simulink model "feedback_plant"  (R2016a)
settings: Solver=FixedStepAuto  StartTime=0.0  StopTime=9660  MaxStep=0.1  RelTol=1e-3
undefined symbols (not defined in the file): sensors
libraries: slrtlib x8, xpcnilib x2, simulink x2
settings Model: ModifiedByFormat=The MathWorks Inc.  Creator=The MathWorks, Inc.  LastModifiedBy=The MathWorks Inc.
settings SolverCC: EnableConcurrentExecution=on
settings DataIOCC: LimitDataPoints=on  SaveFormat=Array
settings OptimizationCC: BlockReduction=off  DefaultParameterBehavior=Inlined  OptimizeBlockIOStorage=off  BufferReuse=off  GlobalBufferReuse=off  ExpressionFolding=off  ExpressionDepthLimit=2147483647  LocalBlockOutputs=off
settings DebuggingCC: UnderspecifiedInitializationDetection=Classic  MergeDetectMultiDrivingBlocksExec=none  SolverPrmCheckMsg=warning  FcnCallInpInsideContextMsg=EnableAllAsWarning  AllowSymbolicDim=off  StateNameClashWarn=warning
settings HardwareCC: ProdBitPerPointer=32  ProdLargestAtomicFloat=None  ProdWordSize=32  ProdLongLongMode=on  ProdHWDeviceType=Generic->32-bit x86 compatible
settings ModelReferenceCC: ModelReferenceNumInstancesAllowed=Single  ModelReferenceMinAlgLoopOccurrences=on  PropagateSignalLabelsOutOfModel=off
settings RTWCC: SystemTargetFile=slrt.tlc  TemplateMakefile=slrt_default_tmf  Description=Simulink Real-Time  RTWVerbose=off
settings ConfigComp: CovModelRefEnable=Off  CovSFcnEnable=off

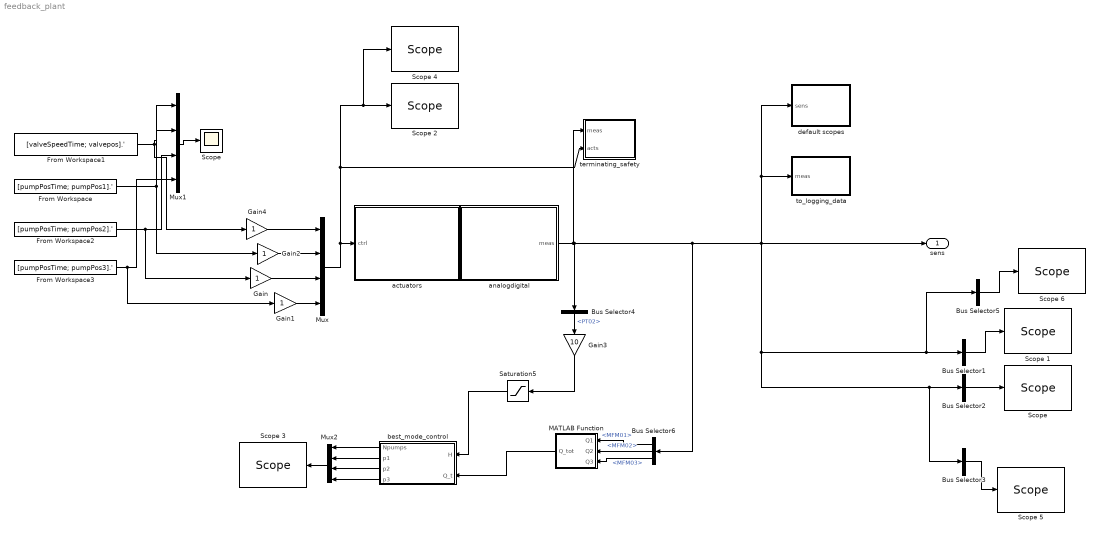
== system feedback_plant ==
  Bus Selector1 : BusSelector  OutputSignals=CV01,DPT01,DPT02,DPT03,MFM01,MFM02,MFM03,PT02  OutputAsBus=on
  Bus Selector2 : BusSelector  OutputSignals=LMGV1,LMGV2,LMGV3,LMGC1,LMGC2,LMGC3,LMGP1,LMGP2,LMGP3  OutputAsBus=on
  Bus Selector3 : BusSelector  OutputSignals=WP01,WP02,WP03  OutputAsBus=on
  Bus Selector4 : BusSelector  OutputSignals=PT02
  Bus Selector5 : BusSelector  OutputSignals=PT02  OutputAsBus=on
  Bus Selector6 : BusSelector  OutputSignals=MFM01,MFM02,MFM03
  From Workspace : FromWorkspace  VariableName=[pumpPosTime; pumpPos1].'  SampleTime=0  Interpolate=off  OutputAfterFinalValue=Holding final value
  From Workspace1 : FromWorkspace  VariableName=[valveSpeedTime; valvepos].'  SampleTime=0  Interpolate=off  OutputAfterFinalValue=Holding final value
  From Workspace2 : FromWorkspace  VariableName=[pumpPosTime; pumpPos2].'  SampleTime=0  Interpolate=off  OutputAfterFinalValue=Holding final value
  From Workspace3 : FromWorkspace  VariableName=[pumpPosTime; pumpPos3].'  SampleTime=0  Interpolate=off  OutputAfterFinalValue=Holding final value
  Gain{,1..2,4} (4 alike) : Gain
  Gain3 : Gain  Gain=10
  MATLAB Function : MATLAB Function  TreatAsAtomicUnit=on
  Mux : Mux
  Mux1 : Mux
  Mux2 : Mux
  Saturation5 : Saturate  UpperLimit=200  LowerLimit=0.001
  Scope : Scope
  "Scope " : slrtlib/Displays and Logging/Scope   scopeno=9  scopetype=Target  autostart=on  viewmode=Numerical  formatstr='%15.6f'  grid=on  ylimits=[0,0]  nosamples=25  noprepostsamples=0  interleave=1  triggermode=FreeRun  triggersignal=1  trigsignalfromport=off  triggerlevel=0.0  triggerslope=Either  triggerscope=1  triggersample=0  filename=data.dat  mode=Lazy  writesize=512  autorestart=off  dynamicfilemode=off  maxwritefilesize=512*1024^2
  Scope 1 : slrtlib/Displays and Logging/Scope   scopeno=10  scopetype=Target  autostart=on  viewmode=Numerical  formatstr='%15.6f'  grid=on  ylimits=[0,0]  nosamples=25  noprepostsamples=0  interleave=1  triggermode=FreeRun  triggersignal=1  trigsignalfromport=off  triggerlevel=0.0  triggerslope=Either  triggerscope=1  triggersample=0  filename=data.dat  mode=Lazy  writesize=512  autorestart=off  dynamicfilemode=off  maxwritefilesize=512*1024^2
  Scope 2 : slrtlib/Displays and Logging/Scope   scopeno=2  scopetype=Host  autostart=on  viewmode=Graphical redraw  formatstr='%15.6f'  grid=on  ylimits=[0,0]  nosamples=250  noprepostsamples=0  interleave=1  triggermode=FreeRun  triggersignal=1  trigsignalfromport=off  triggerlevel=0.0  triggerslope=Either  triggerscope=1  triggersample=0  filename=data.dat  mode=Lazy  writesize=512  autorestart=off  dynamicfilemode=off  maxwritefilesize=512*1024^2
  Scope 3 : slrtlib/Displays and Logging/Scope   scopeno=3  scopetype=Host  autostart=on  viewmode=Graphical redraw  formatstr='%15.6f'  grid=on  ylimits=[0,0]  nosamples=250  noprepostsamples=0  interleave=1  triggermode=FreeRun  triggersignal=1  trigsignalfromport=off  triggerlevel=0.0  triggerslope=Either  triggerscope=1  triggersample=0  filename=data.dat  mode=Lazy  writesize=512  autorestart=off  dynamicfilemode=off  maxwritefilesize=512*1024^2
  Scope 4 : slrtlib/Displays and Logging/Scope   scopeno=8  scopetype=Target  autostart=on  viewmode=Numerical  formatstr='%15.6f'  grid=on  ylimits=[0,0]  nosamples=25  noprepostsamples=0  interleave=1  triggermode=FreeRun  triggersignal=1  trigsignalfromport=off  triggerlevel=0.0  triggerslope=Either  triggerscope=1  triggersample=0  filename=data.dat  mode=Lazy  writesize=512  autorestart=off  dynamicfilemode=off  maxwritefilesize=512*1024^2
  Scope 5 : slrtlib/Displays and Logging/Scope   scopeno=11  scopetype=Target  autostart=on  viewmode=Numerical  formatstr='%15.6f'  grid=on  ylimits=[0,0]  nosamples=25  noprepostsamples=0  interleave=1  triggermode=FreeRun  triggersignal=1  trigsignalfromport=off  triggerlevel=0.0  triggerslope=Either  triggerscope=1  triggersample=0  filename=data.dat  mode=Lazy  writesize=512  autorestart=off  dynamicfilemode=off  maxwritefilesize=512*1024^2
  Scope 6 : slrtlib/Displays and Logging/Scope   scopeno=4  scopetype=Target  autostart=on  viewmode=Graphical sliding  formatstr='%15.6f'  grid=on  ylimits=[0,0]  nosamples=100  noprepostsamples=0  interleave=1  triggermode=FreeRun  triggersignal=1  trigsignalfromport=off  triggerlevel=0.0  triggerslope=Either  triggerscope=1  triggersample=0  filename=data.dat  mode=Lazy  writesize=512  autorestart=off  dynamicfilemode=off  maxwritefilesize=512*1024^2
  actuators : Subsystem  mask{actuators_list={'CV03', 'CV05'}, subsystem=[3,1]}
      mask init:
      | %%Get analog channels
      | actuators = evalin('base','actuators');
      | 
      | subsystem = sprintf('[%d,%d]', subsystem(1), subsystem(2));
      | 
      | %actuators = actuators(strcmp(subsystem,{actuators.PCIslot}));
      | 
      | src_block = find_system(gcb, 'LookUnderMasks', 'on','Name', 'DA_sink');
      | maskObj = Simulink.Mask.get(src_block{1});
      | 
      | if(isempty(actuators))
      |    error('There are no analog outputs in the given card'); 
      | end
      | 
      | maskObj.Parameters(1,5).Value = subsystem;
      | maskObj.Parameters(1,1).Value = mat2str([actuators.Channel]+1);
      | Simulink.Block.eval(src_block{1});
      | 
      | %Find block
      | transform_blk = find_system(gcb, 'LookUnderMasks', 'on','Name', 'transform');
      | 
      | outputnames = {actuators.Name};
      | outputs = strjoin(outputnames,',');
      | 
      | sigcount = numel(outputnames);
      | sigstring = num2str(sigcount);
      | 
      | %Transform block
      | transform_blk = find_system(gcb, 'LookUnderMasks', 'on','Name', 'transform');
      | lines{1}=['function [' outputs ']  = fcn(u,gain,offset)'];
      | lines{2}='   y = u.*gain-offset;';
      | for i=1:numel(outputnames)
      |    %start at 4
      |    lines{2+i} = [ outputnames{i} ' = y(' num2str(i) ');'];
      | end
      | outputscript = strjoin(lines,'\n');
      | matlabfunctionfromstring(transform_blk{1}, outputscript);
      | Simulink.Block.eval(transform_blk{1});
      | 
      | %Delete lines
      | connections = find_system(gcb,'findall','on','LookUnderMasks', 'on','SearchDepth', 1,'type','line');
      | delete_line(connections);
      | 
      | for i=1:numel(outputnames)
      |    add_line(gcb,['transform/' num2str(i) ],['DA_sink/' num2str(i)],'autorouting','on');
      | end
      | 
      | %Transform block
      | add_line(gcb,'ctrl/1','transform/1','autorouting','on')
      | add_line(gcb,'gain/1','transform/2','autorouting','on')
      | add_line(gcb,'offset/1','transform/3','autorouting','on')
      | 
      | gain = [actuators.Gain]';
      | offset = [actuators.Offset]';
  analogdigital : Subsystem  mask{gain=[sensors.Gain], offset=[sensors.Offset]}
      mask init:
      | %%Get analog channels
      | sensors = evalin('base','sensors');
      | 
      | %subsystem = sprintf('[%d,%d]', subsystem(1), subsystem(2));
      | 
      | %analogin = sensors(strcmp(subsystem,{sensors.PCIslot})&(strcmp('VI|0-10V',{sensors.Type})|strcmp('VI|2-10V',{sensors.Type})|strcmp('CI|4-20mA',{sensors.Type})));
      | if ~isempty(sensors)
      | %    disp(['PCI slot ' subsystem ' loading']);
      | else
      |     error('There are no analog inputs in the given card'); 
      | end
      | 
      | 
      | %%Find source (ADC) block
      | src_block = find_system(gcb, 'LookUnderMasks', 'on','Name', 'src');
      | maskObj = Simulink.Mask.get(src_block{1});
      | 
      | %maskObj.Parameters(1,6).Value = subsystem;
      | maskObj.Parameters(1,1).Value = mat2str([sensors.Channel]+1);
      | Simulink.Block.eval(src_block{1});
      | 
      | %Find block
      | transform_blk = find_system(gcb, 'LookUnderMasks', 'on','Name', 'transform');
      | 
      | outputnames = {sensors.Name};
      | outputs = strjoin(outputnames,',');
      | 
      | sigcount = numel(outputnames);
      | sigstring = num2str(sigcount);
      | 
      | %Transform block
      | transform_blk = find_system(gcb, 'LookUnderMasks', 'on','Name', 'transform');
      | lines{1}=['function [' outputs ']  = fcn(u,gain,offset)'];
      | lines{2}='   y = u(:).*gain(:)-offset(:);';
      | for i=1:numel(outputnames)
      |    %start at 4
      |    lines{2+i} = [ outputnames{i} ' = y(' num2str(i) ');'];
      | end
      | outputscript = strjoin(lines,'\n');
      | matlabfunctionfromstring(transform_blk{1}, outputscript);
      | Simulink.Block.eval(transform_blk{1});
      | 
      | %Delete lines
      | connections = find_system(gcb,'findall','on','LookUnderMasks', 'on','SearchDepth', 1,'type','line');
      | delete_line(connections);
      | 
      | %Mux block
      | mux_blk = find_system(gcb, 'LookUnderMasks', 'on','Name', 'mux');
      | set_param(mux_blk{1},'Inputs', sigstring);
      | Simulink.Block.eval(mux_blk{1});
      | 
      | %Bus block
      | bus_blk = find_system(gcb, 'LookUnderMasks', 'on','Name', 'bus');
      | set_param(bus_blk{1},'Inputs', sigstring);
      | Simulink.Block.eval(bus_blk{1});
      | 
      | for i=1:numel(outputnames)
      |    add_line(gcb,['src/' num2str(i) ],['mux/' num2str(i)],'autorouting','on');
      |    add_line(gcb,['transform/' num2str(i) ],['bus/' num2str(i)],'autorouting','on');
      | end
      | 
      | %Lines to bus block
      | p = get_param(transform_blk, 'PortHandles');
      | l = get_param(p{1}.Outport,'Line');
      | 
      | for i=1:numel(outputnames)
      |    set_param(l{i},'Name',outputnames{i}) 
      | end
      | 
      | %Transform block
      | add_line(gcb,'mux/1','transform/1','autorouting','on')
      | add_line(gcb,'bus/1','meas/1','autorouting','on')
  best_mode_control : Subsystem
  default scopes : Subsystem
  terminating_safety : Subsystem
      mask init:
      | str1 = evalin('base', 'strjoin({sensors.Name},''/'')');
      | sensnames = uint8(str1);
  to_logging_data : Subsystem
  sens : Outport
  wires:
  Mux/1 -> actuators/1(ctrl), terminating_safety/2(acts), Scope 4/1, Scope 2/1
  Bus Selector2/1 -> "Scope "/1
  Bus Selector1/1 -> Scope 1/1
  Mux1/1 -> Scope/1
  From Workspace1/1 -> Mux1/1, Gain4/1
  From Workspace/1 -> Gain2/1, Mux1/2
  Bus Selector3/1 -> Scope 5/1
  Bus Selector5/1 -> Scope 6/1
  Gain/1 -> Mux/3
  Gain1/1 -> Mux/4
  Gain2/1 -> Mux/2
  analogdigital/1(meas) -> terminating_safety/1(meas), Bus Selector6/1, default scopes/1(sens), to_logging_data/1(meas), Bus Selector5/1, Bus Selector1/1, Bus Selector3/1, Bus Selector2/1, sens/1, Bus Selector4/1
  Bus Selector6/2 -> MATLAB Function/2(Q2)  "<MFM02>"
  Bus Selector6/1 -> MATLAB Function/1(Q1)  "<MFM01>"
  Bus Selector6/3 -> MATLAB Function/3(Q3)  "<MFM03>"
  MATLAB Function/1(Q_tot) -> best_mode_control/2(Q_t)
  Bus Selector4/1 -> Gain3/1  "<PT02>"
  Gain3/1 -> Saturation5/1
  Mux2/1 -> Scope 3/1
  best_mode_control/1(Npumps) -> Mux2/1
  best_mode_control/2(p1) -> Mux2/2
  best_mode_control/3(p2) -> Mux2/3
  best_mode_control/4(p3) -> Mux2/4
  From Workspace2/1 -> Gain/1, Mux1/3
  From Workspace3/1 -> Gain1/1, Mux1/4
  Saturation5/1 -> best_mode_control/1(H)
  Gain4/1 -> Mux/1

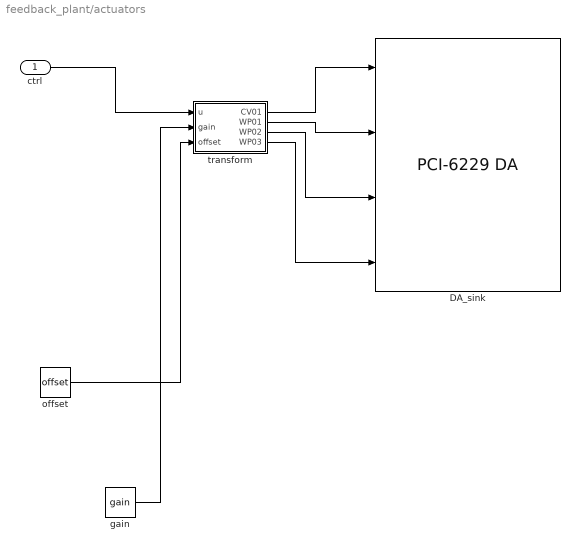
== system feedback_plant/actuators ==
  ctrl : Inport
  DA_sink : xpcnilib/D//A/M Series/PCI-6229 DA  channel=[4 1 2 3]  reset=[1]  initValue=[0]  sampletime=0.01  slot=[3,1]
  gain : Constant  Value=gain
  offset : Constant  Value=offset
  transform : MATLAB Function  TreatAsAtomicUnit=on
  wires:
  transform/1(CV01) -> DA_sink/1
  transform/2(WP01) -> DA_sink/2
  transform/3(WP02) -> DA_sink/3
  transform/4(WP03) -> DA_sink/4
  ctrl/1 -> transform/1(u)
  gain/1 -> transform/2(gain)
  offset/1 -> transform/3(offset)

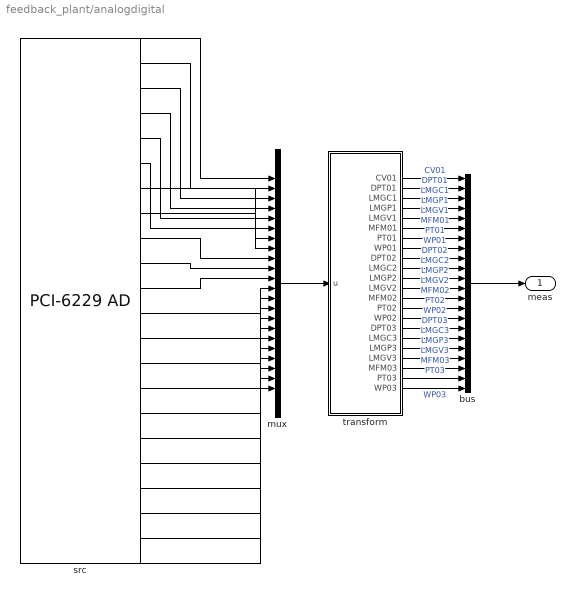
== system feedback_plant/analogdigital ==
  bus : BusCreator  Inputs=22
  mux : Mux  Inputs=22
  src : xpcnilib/A//D/M Series/PCI-6229 AD  channel=[4 17 5 11 8 21 24 1 18 6 12 9 22 25 2 19 7 13 10 23 26 3]  range=[10]  coupling=[0]  scantime=5e-6  sampletime=0.01  slot=[3,1]
  transform : MATLAB Function  TreatAsAtomicUnit=on
  meas : Outport
  wires:
  src/1 -> mux/1
  transform/1(CV01) -> bus/1  "CV01"
  src/2 -> mux/2
  transform/2(DPT01) -> bus/2  "DPT01"
  src/3 -> mux/3
  transform/3(LMGC1) -> bus/3  "LMGC1"
  src/4 -> mux/4
  transform/4(LMGP1) -> bus/4  "LMGP1"
  src/5 -> mux/5
  transform/5(LMGV1) -> bus/5  "LMGV1"
  src/6 -> mux/6
  transform/6(MFM01) -> bus/6  "MFM01"
  src/7 -> mux/7
  transform/7(PT01) -> bus/7  "PT01"
  src/8 -> mux/8
  transform/8(WP01) -> bus/8  "WP01"
  src/9 -> mux/9
  transform/9(DPT02) -> bus/9  "DPT02"
  src/10 -> mux/10
  transform/10(LMGC2) -> bus/10  "LMGC2"
  src/11 -> mux/11
  transform/11(LMGP2) -> bus/11  "LMGP2"
  src/12 -> mux/12
  transform/12(LMGV2) -> bus/12  "LMGV2"
  src/13 -> mux/13
  transform/13(MFM02) -> bus/13  "MFM02"
  src/14 -> mux/14
  transform/14(PT02) -> bus/14  "PT02"
  src/15 -> mux/15
  transform/15(WP02) -> bus/15  "WP02"
  src/16 -> mux/16
  transform/16(DPT03) -> bus/16  "DPT03"
  src/17 -> mux/17
  transform/17(LMGC3) -> bus/17  "LMGC3"
  src/18 -> mux/18
  transform/18(LMGP3) -> bus/18  "LMGP3"
  src/19 -> mux/19
  transform/19(LMGV3) -> bus/19  "LMGV3"
  src/20 -> mux/20
  transform/20(MFM03) -> bus/20  "MFM03"
  src/21 -> mux/21
  transform/21(PT03) -> bus/21  "PT03"
  src/22 -> mux/22
  transform/22(WP03) -> bus/22  "WP03"
  mux/1 -> transform/1(u)
  bus/1 -> meas/1

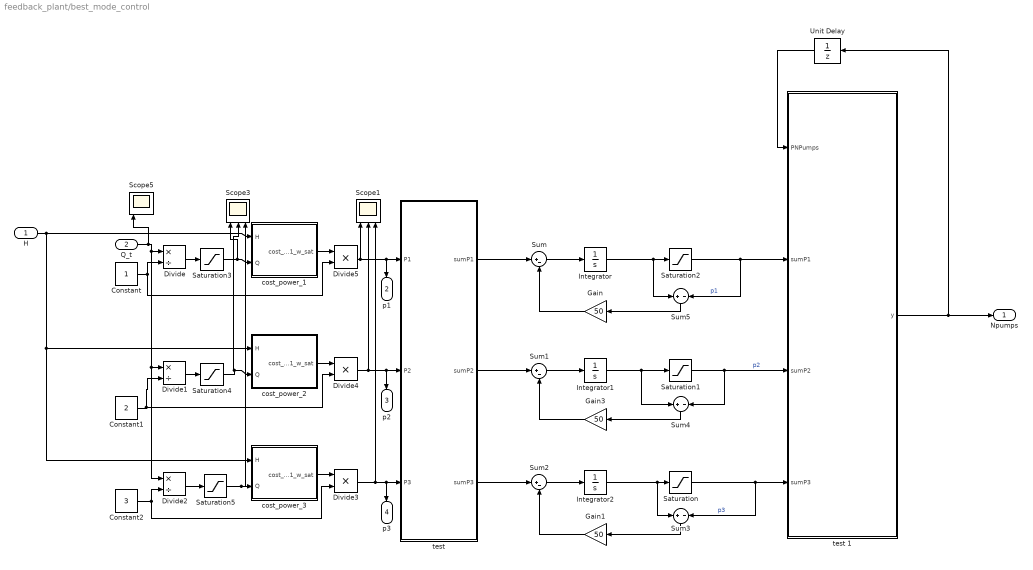
== system feedback_plant/best_mode_control ==
  H : Inport
  Q_t : Inport  Port=2
  Constant : Constant
  Constant1 : Constant  Value=2
  Constant2 : Constant  Value=3
  Divide : Product  Inputs=*/
  Divide1 : Product  Inputs=*/
  Divide2 : Product  Inputs=*/
  Divide3 : Product  Inputs=**
  Divide4 : Product  Inputs=**
  Divide5 : Product  Inputs=**
  Gain : Gain  Gain=50
  Gain1 : Gain  Gain=50
  Gain3 : Gain  Gain=50
  Integrator : Integrator  UpperSaturationLimit=100  LowerSaturationLimit=-100
  Integrator1 : Integrator  UpperSaturationLimit=100  LowerSaturationLimit=-100
  Integrator2 : Integrator  UpperSaturationLimit=100  LowerSaturationLimit=-100
  Saturation : Saturate  UpperLimit=200  LowerLimit=-200
  Saturation1 : Saturate  UpperLimit=200  LowerLimit=-200
  Saturation2 : Saturate  UpperLimit=200  LowerLimit=-200
  Saturation3 : Saturate  UpperLimit=15  LowerLimit=0
  Saturation4 : Saturate  UpperLimit=15  LowerLimit=0
  Saturation5 : Saturate  UpperLimit=15  LowerLimit=0
  Scope1 : Scope  NumInputPorts=3
  Scope3 : Scope  NumInputPorts=3
  Scope5 : Scope  NumInputPorts=3
  Sum : Sum  Inputs=|+-
  Sum1 : Sum  Inputs=|+-
  Sum2 : Sum  Inputs=|+-
  Sum3 : Sum  Inputs=+|-
  Sum4 : Sum  Inputs=+|-
  Sum5 : Sum  Inputs=+|-
  Unit Delay : UnitDelay  InitialCondition=1  SampleTime=-1
  cost_power_1 : MATLAB Function  TreatAsAtomicUnit=on
  cost_power_2 : MATLAB Function  TreatAsAtomicUnit=on
  cost_power_3 : MATLAB Function  TreatAsAtomicUnit=on
  "test " : MATLAB Function  TreatAsAtomicUnit=on
  test 1 : MATLAB Function  TreatAsAtomicUnit=on
  Npumps : Outport
  p1 : Outport  Port=2
  p2 : Outport  Port=3
  p3 : Outport  Port=4
  wires:
  test 1/1(y) -> Unit Delay/1, Npumps/1
  H/1 -> cost_power_1/1(H), cost_power_2/1(H), cost_power_3/1(H)
  Q_t/1 -> Scope5/1, Divide2/1, Divide1/1, Divide/1
  Divide/1 -> Saturation3/1
  Constant/1 -> Divide5/2, Divide/2
  Constant1/1 -> Divide1/2, Divide4/2
  Divide1/1 -> Saturation4/1
  Constant2/1 -> Divide3/2, Divide2/2
  Divide2/1 -> Saturation5/1
  Divide5/1 -> Scope1/1, p1/1, "test "/1(P1)
  Divide3/1 -> p3/1, "test "/3(P3), Scope1/3
  Sum1/1 -> Integrator1/1
  Integrator/1 -> Saturation2/1, Sum5/1
  Integrator1/1 -> Saturation1/1, Sum4/1
  cost_power_3/1(cost_power_1_w_sat) -> Divide3/1
  cost_power_2/1(cost_power_1_w_sat) -> Divide4/1
  cost_power_1/1(cost_power_1_w_sat) -> Divide5/1
  Integrator2/1 -> Sum3/1, Saturation/1
  Gain1/1 -> Sum2/2
  "test "/3(sumP3) -> Sum2/1
  "test "/2(sumP2) -> Sum1/1
  Sum3/1 -> Gain1/1
  Sum/1 -> Integrator/1
  Sum5/1 -> Gain/1
  Sum2/1 -> Integrator2/1
  Saturation/1 -> Sum3/2, test 1/4(sumP3)  "p3"
  Saturation1/1 -> test 1/3(sumP2), Sum4/2  "p2"
  Saturation2/1 -> Sum5/2, test 1/2(sumP1)  "p1"
  Sum4/1 -> Gain3/1
  Gain3/1 -> Sum1/2
  Unit Delay/1 -> test 1/1(PNPumps)
  Saturation3/1 -> Scope3/1, cost_power_1/2(Q)
  Saturation4/1 -> cost_power_2/2(Q), Scope3/2
  Saturation5/1 -> Scope3/3, cost_power_3/2(Q)
  "test "/1(sumP1) -> Sum/1
  Gain/1 -> Sum/2
  Divide4/1 -> Scope1/2, p2/1, "test "/2(P2)

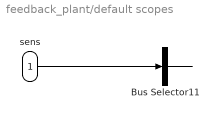
== system feedback_plant/default scopes ==
  sens : Inport
  Bus Selector11 : BusSelector  OutputSignals=CV01,DPT01,LMGC1  OutputAsBus=on
  wires:
  sens/1 -> Bus Selector11/1
  Bus Selector11/1 -> ?

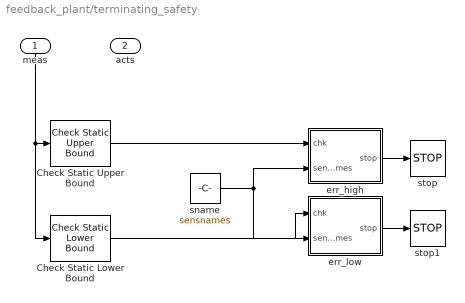
== system feedback_plant/terminating_safety ==
  meas : Inport
  acts : Inport  Port=2
  Check Static Lower Bound : simulink/Model Verification/Check Static  Lower Bound  Description=[sensors.MinOp]-([sensors.MaxOp]-[sensors.MinOp])*0.05 <= u  min=[sensors.MinOp]-([sensors.MaxOp]-[sensors.MinOp])*0.05  min_included=on  enabled=on  stopWhenAssertionFail=off  export=on  icon=graphic
  Check Static Upper Bound : simulink/Model Verification/Check Static  Upper Bound  Description=u <= [sensors.MaxOp]+([sensors.MaxOp]-[sensors.MinOp])*0.05  max=[sensors.MaxOp]+([sensors.MaxOp]-[sensors.MinOp])*0.05  max_included=on  enabled=on  stopWhenAssertionFail=off  export=on  icon=graphic
  err_high : MATLAB Function  TreatAsAtomicUnit=on
  err_low : MATLAB Function  TreatAsAtomicUnit=on
  sname : Constant  Value=sensnames
  stop : Stop
  stop1 : Stop
  wires:
  Check Static Upper Bound/1 -> err_high/1(chk)
  Check Static Lower Bound/1 -> err_low/1(chk)
  sname/1 -> err_high/2(sensnames), err_low/2(sensnames)
  err_high/1(stop) -> stop/1
  err_low/1(stop) -> stop1/1
  meas/1 -> Check Static Lower Bound/1, Check Static Upper Bound/1

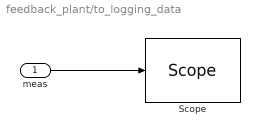
== system feedback_plant/to_logging_data ==
  meas : Inport
  "Scope " : slrtlib/Displays and Logging/Scope   scopeno=1  scopetype=Host  autostart=on  viewmode=Graphical redraw  formatstr='%15.6f'  grid=on  ylimits=[0,0]  nosamples=250  noprepostsamples=0  interleave=1  triggermode=FreeRun  triggersignal=1  trigsignalfromport=off  triggerlevel=0.0  triggerslope=Either  triggerscope=1  triggersample=0  filename=data.dat  mode=Lazy  writesize=512  autorestart=off  dynamicfilemode=off  maxwritefilesize=512*1024^2
  wires:
  meas/1 -> "Scope "/1

== matlab function feedback_plant/actuators/transform ==
  data: u input; CV01 output; gain input; offset input; WP01 output; WP02 output; WP03 output
function [CV01,WP01,WP02,WP03]  = fcn(u,gain,offset)
   y = u.*gain-offset;
CV01 = y(1);
WP01 = y(2);
WP02 = y(3);
WP03 = y(4);

== matlab function feedback_plant/analogdigital/transform ==
  data: CV01 output size=1; u input; gain parameter; offset parameter; DPT01 output; LMGC1 output; LMGP1 output; LMGV1 output; MFM01 output; PT01 output; WP01 output; DPT02 output; LMGC2 output; LMGP2 output; LMGV2 output; MFM02 output; PT02 output; WP02 output; DPT03 output; LMGC3 output; LMGP3 output; LMGV3 output; MFM03 output; PT03 output; WP03 output
function [CV01,DPT01,LMGC1,LMGP1,LMGV1,MFM01,PT01,WP01,DPT02,LMGC2,LMGP2,LMGV2,MFM02,PT02,WP02,DPT03,LMGC3,LMGP3,LMGV3,MFM03,PT03,WP03]  = fcn(u,gain,offset)
   y = u(:).*gain(:)-offset(:);
CV01 = y(1);
DPT01 = y(2);
LMGC1 = y(3);
LMGP1 = y(4);
LMGV1 = y(5);
MFM01 = y(6);
PT01 = y(7);
WP01 = y(8);
DPT02 = y(9);
LMGC2 = y(10);
LMGP2 = y(11);
LMGV2 = y(12);
MFM02 = y(13);
PT02 = y(14);
WP02 = y(15);
DPT03 = y(16);
LMGC3 = y(17);
LMGP3 = y(18);
LMGV3 = y(19);
MFM03 = y(20);
PT03 = y(21);
WP03 = y(22);

== matlab function feedback_plant/MATLAB Function ==
  data: Q1 input; Q_tot output; Q2 input; Q3 input
function Q_tot = fcn(Q1, Q2, Q3)

Q_tot = ((Q1 + Q2 + Q3) *60 * 60)/1000;

== matlab function feedback_plant/terminating_safety/err_high ==
  data: chk input; sensnames input uint8; stop output
function stop  = fcn(chk, sensnames)
%#codegen
%test = char(sensnames.');
test = sensnames.';
k = find(test == 47);
k = [0 k];
k = [k numel(test)];
stop = 0;
for i = 1:numel(chk)
    if chk(i) == 0
        str = char(test(k(i)+1:k(i+1)-1));
        Error = [str ': VALUE TOO HIGH ']
        coder.ceval('printf', ['%s' 10 0], Error);
        stop = stop+1;
    end
end

== matlab function feedback_plant/terminating_safety/err_low ==
  data: chk input; sensnames input uint8; stop output
function stop  = fcn(chk, sensnames)
%#codegen
test = char(sensnames.');
k = strfind(test, '/');
k = [0 k];
k = [k numel(sensnames)];
stop = 0;
for i = 1:numel(chk)
    if chk(i) == 0
        str = char(test(k(i)+1:k(i+1)-1));
        Error = [str ': VALUE TOO LOW']
        coder.ceval('printf', ['%s' 10 0], Error);
        stop = stop+1;
    end
end

== matlab function feedback_plant/best_mode_control/cost_power_1 ==
  data: cost_power_1_w_sat output; H input; Q input
function cost_power_1_w_sat = cost_power_1(H,Q)
%#codegen

%    This function was generated by the Symbolic Math Toolbox version 7.0.
%    14-Oct-2016 11:25:59

t2 = H.^2;
t3 = Q.^2;
t4 = H.*1.396903852036515e2;
t5 = Q.*3.495225250698616e1;
t6 = H.*t3.*1.223287779152999e-1;
t7 = Q.*t2.*1.66325485327369e-1;
t8 = H.*t2.*2.226602402994795e-2;
t9 = t3.*3.770314092453583e1;
t13 = t2.*2.5749360250113;
t14 = Q.*t3.*1.742768641280902;
t15 = H.*Q.*1.124558547771882e1;
t10 = t4+t5+t6+t7+t8+t9-t13-t14-t15+5.473012823773138e2;
t11 = t10;
t12 = max([t11,0.0]);
t16 = H.^1.386296711773041;
t17 = t16.*2.358991511181789;
t18 = Q.^2.776519861495102;
t19 = t18.*1.317701188625407;
t20 = H.*Q.*2.773249178787912;
t21 = t17+t19+t20+2.725420441582497e1;
cost_power_1_w_sat = double(((t12 < 3.6e2) || (1.8e3 < t21)) || (3.6e3 < t12)).*5.0e4+t21.*double(((3.6e2 <= t12) && (t21 <= 1.8e3)) && (t12 <= 3.6e3));

== matlab function feedback_plant/best_mode_control/test  ==
  data: sumP1 output; P1 input; P2 input; P3 input; sumP2 output; sumP3 output
function [sumP1, sumP2, sumP3] = cost_power_1(P1, P2, P3)
sumP1 = min(P2,P3) - P1;
sumP2 = min(P1,P3) - P2;
sumP3 = min(P1,P2) - P3;

== matlab function feedback_plant/best_mode_control/cost_power_2 ==
  data: cost_power_1_w_sat output; H input; Q input
function cost_power_1_w_sat = cost_power_2(H,Q)
%#codegen

%    This function was generated by the Symbolic Math Toolbox version 7.0.
%    14-Oct-2016 11:25:59

t2 = H.^2;
t3 = Q.^2;
t4 = H.*1.396903852036515e2;
t5 = Q.*3.495225250698616e1;
t6 = H.*t3.*1.223287779152999e-1;
t7 = Q.*t2.*1.66325485327369e-1;
t8 = H.*t2.*2.226602402994795e-2;
t9 = t3.*3.770314092453583e1;
t13 = t2.*2.5749360250113;
t14 = Q.*t3.*1.742768641280902;
t15 = H.*Q.*1.124558547771882e1;
t10 = t4+t5+t6+t7+t8+t9-t13-t14-t15+5.473012823773138e2;
t11 = t10;
t12 = max([t11,0.0]);
t16 = H.^1.386296711773041;
t17 = t16.*2.358991511181789;
t18 = Q.^2.776519861495102;
t19 = t18.*1.317701188625407;
t20 = H.*Q.*2.773249178787912;
t21 = t17+t19+t20+2.725420441582497e1;
cost_power_1_w_sat = double(((t12 < 3.6e2) || (1.8e3 < t21)) || (3.6e3 < t12)).*5.0e4+t21.*double(((3.6e2 <= t12) && (t21 <= 1.8e3)) && (t12 <= 3.6e3));

== matlab function feedback_plant/best_mode_control/cost_power_3 ==
  data: cost_power_1_w_sat output; H input; Q input
function cost_power_1_w_sat = cost_power_3(H,Q)
%#codegen

%    This function was generated by the Symbolic Math Toolbox version 7.0.
%    14-Oct-2016 11:25:59

t2 = H.^2;
t3 = Q.^2;
t4 = H.*1.396903852036515e2;
t5 = Q.*3.495225250698616e1;
t6 = H.*t3.*1.223287779152999e-1;
t7 = Q.*t2.*1.66325485327369e-1;
t8 = H.*t2.*2.226602402994795e-2;
t9 = t3.*3.770314092453583e1;
t13 = t2.*2.5749360250113;
t14 = Q.*t3.*1.742768641280902;
t15 = H.*Q.*1.124558547771882e1;
t10 = t4+t5+t6+t7+t8+t9-t13-t14-t15+5.473012823773138e2;
t11 = t10;
t12 = max([t11,0.0]);
t16 = H.^1.386296711773041;
t17 = t16.*2.358991511181789;
t18 = Q.^2.776519861495102;
t19 = t18.*1.317701188625407;
t20 = H.*Q.*2.773249178787912;
t21 = t17+t19+t20+2.725420441582497e1;
cost_power_1_w_sat = double(((t12 < 3.6e2) || (1.8e3 < t21)) || (3.6e3 < t12)).*5.0e4+t21.*double(((3.6e2 <= t12) && (t21 <= 1.8e3)) && (t12 <= 3.6e3));

== matlab function feedback_plant/best_mode_control/test 1 ==
  data: PNPumps input; y output; sumP1 input; sumP2 input; sumP3 input
function y = cost_power_1(PNPumps,sumP1, sumP2, sumP3)
powerVector = [sumP1, sumP2, sumP3];
[~,Npumps] = max([sumP1, sumP2, sumP3]);
if Npumps == PNPumps
    y = Npumps;
else 
    if abs(powerVector(Npumps) - powerVector(PNPumps)) > 10
        y = Npumps;
    else
        y = PNPumps;
    end
    
end
